simulink subsystem "Plant_d"  (R2024b)
settings: Solver=VariableStepAuto  StartTime=0.0  StopTime=10.0  RelTol=1e-3
undefined symbols (not defined in the file): body, DiscIntNeverNeededParam, wheels
settings Model: Creator=Marij  LastModifiedBy=marijn

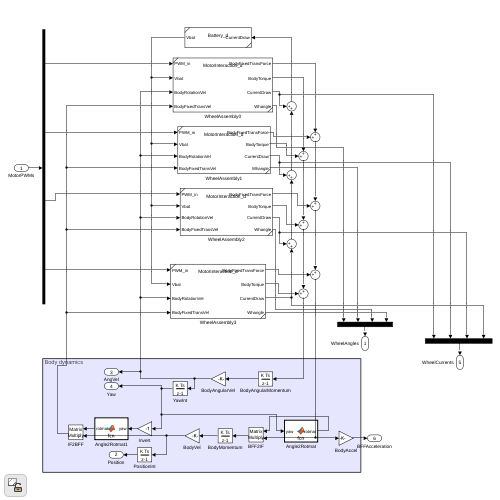
[thumbnail: Simulink's stored preview of the top-level diagram]
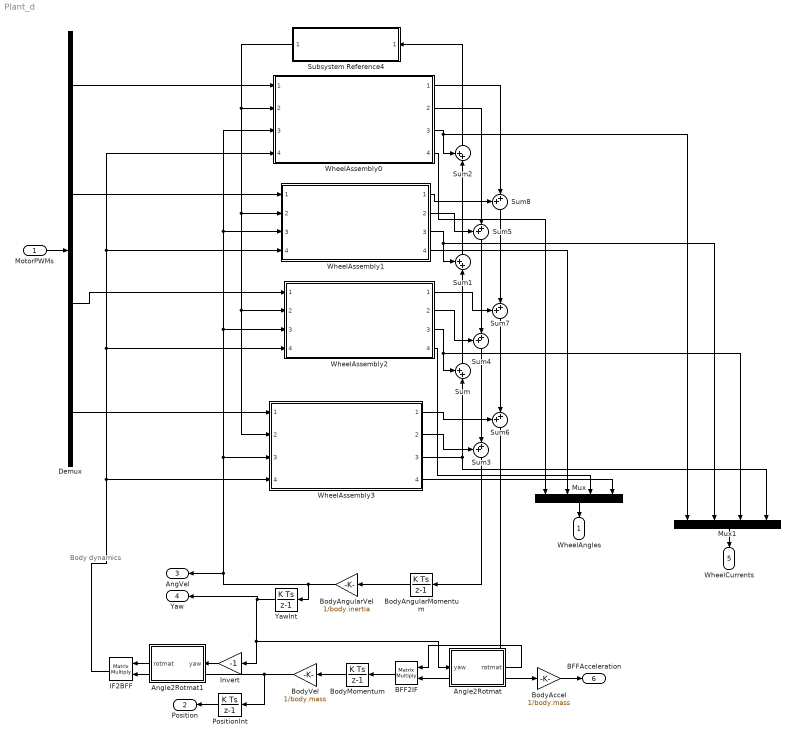
== system Plant_d ==
  note: Body dynamics
  MotorPWMs : Inport  PortDimensions=4
  Angle2Rotmat : MATLAB Function  TreatAsAtomicUnit=on
  Angle2Rotmat1 : MATLAB Function  TreatAsAtomicUnit=on
  BFF2IF : Product  Multiplication=Matrix(*)
  BodyAccel : Gain  Gain=1/body.mass
  BodyAngularMomentum : DiscreteIntegrator  SampleTime=0.0100000000000000002  ICPrevOutput=DiscIntNeverNeededParam  ICPrevScaledInput=DiscIntNeverNeededParam  mask(DiscretizedDiscreteIntegrator){}
      mask init:
      | %zoh
  BodyAngularVel : Gain  Gain=1/body.inertia
  BodyMomentum : DiscreteIntegrator  SampleTime=0.0100000000000000002  ICPrevOutput=DiscIntNeverNeededParam  ICPrevScaledInput=DiscIntNeverNeededParam  mask(DiscretizedDiscreteIntegrator){}
      mask init:
      | %zoh
  BodyVel : Gain  Gain=1/body.mass
  Demux : Demux
  IF2BFF : Product  Multiplication=Matrix(*)
  Invert : Gain  Gain=-1
  Mux : Mux
  Mux1 : Mux
  PositionInt : DiscreteIntegrator  SampleTime=0.0100000000000000002  ICPrevOutput=DiscIntNeverNeededParam  ICPrevScaledInput=DiscIntNeverNeededParam  mask(DiscretizedDiscreteIntegrator){}
      mask init:
      | %zoh
  Subsystem Reference4 : Subsystem  ReferencedSubsystem=Battery_d
  Sum{,1..8} (9 alike) : Sum  Inputs=++|
  WheelAssembly0 : Subsystem  ReferencedSubsystem=MotorInteraction_d  whangle=wheels.angles(1)
  WheelAssembly1 : Subsystem  ReferencedSubsystem=MotorInteraction_d  whangle=wheels.angles(2)
  WheelAssembly2 : Subsystem  ReferencedSubsystem=MotorInteraction_d  whangle=wheels.angles(3)
  WheelAssembly3 : Subsystem  ReferencedSubsystem=MotorInteraction_d  whangle=wheels.angles(4)
  YawInt : DiscreteIntegrator  SampleTime=0.0100000000000000002  ICPrevOutput=DiscIntNeverNeededParam  ICPrevScaledInput=DiscIntNeverNeededParam  mask(DiscretizedDiscreteIntegrator){}
      mask init:
      | %zoh
  WheelAngles : Outport  Unit=rad  PortDimensions=4
  Position : Outport  Port=2  Unit=m  PortDimensions=2
  AngVel : Outport  Port=3  Unit=rad/s  PortDimensions=1
  Yaw : Outport  Port=4  Unit=rad  PortDimensions=1
  WheelCurrents : Outport  Port=5  Unit=A  PortDimensions=4
  BFFAcceleration : Outport  Port=6
  wires:
  YawInt/1 -> Yaw/1, Angle2Rotmat/1(yaw), Invert/1
  BodyAccel/1 -> BFFAcceleration/1
  Subsystem Reference4/1 -> WheelAssembly0/2, WheelAssembly1/2, WheelAssembly2/2, WheelAssembly3/2
  Mux1/1 -> WheelCurrents/1
  Sum6/1 -> BodyAccel/1, BFF2IF/2
  Sum2/1 -> Subsystem Reference4/1
  WheelAssembly3/4 -> Mux/4
  WheelAssembly0/4 -> Mux/1
  Sum3/1 -> BodyAngularMomentum/1
  Angle2Rotmat1/1(rotmat) -> IF2BFF/1
  BodyMomentum/1 -> BodyVel/1
  BodyVel/1 -> PositionInt/1, IF2BFF/2
  IF2BFF/1 -> WheelAssembly2/4, WheelAssembly1/4, WheelAssembly0/4, WheelAssembly3/4
  Mux/1 -> WheelAngles/1
  BodyAngularMomentum/1 -> BodyAngularVel/1
  WheelAssembly2/2 -> Sum4/1
  WheelAssembly2/4 -> Mux/3
  WheelAssembly0/3 -> Mux1/1, Sum2/1
  PositionInt/1 -> Position/1
  MotorPWMs/1 -> Demux/1
  Sum/1 -> Sum1/2
  WheelAssembly1/3 -> Mux1/2, Sum1/1
  Sum1/1 -> Sum2/2
  Demux/3 -> WheelAssembly2/1
  Demux/4 -> WheelAssembly3/1
  WheelAssembly3/3 -> Mux1/4, Sum/2
  Demux/1 -> WheelAssembly0/1
  BodyAngularVel/1 -> YawInt/1, AngVel/1, WheelAssembly2/3, WheelAssembly1/3, WheelAssembly0/3, WheelAssembly3/3
  Sum8/1 -> Sum7/2
  Sum4/1 -> Sum3/2
  WheelAssembly1/4 -> Mux/2
  Angle2Rotmat/1(rotmat) -> BFF2IF/1
  BFF2IF/1 -> BodyMomentum/1
  WheelAssembly2/3 -> Mux1/3, Sum/1
  WheelAssembly1/1 -> Sum8/1
  WheelAssembly3/2 -> Sum3/1
  Invert/1 -> Angle2Rotmat1/1(yaw)
  WheelAssembly1/2 -> Sum5/1
  WheelAssembly0/1 -> Sum8/2
  Demux/2 -> WheelAssembly1/1
  WheelAssembly3/1 -> Sum6/1
  WheelAssembly2/1 -> Sum7/1
  Sum7/1 -> Sum6/2
  Sum5/1 -> Sum4/2
  WheelAssembly0/2 -> Sum5/2

== matlab function Plant_d/Angle2Rotmat ==
  data: yaw input; rotmat output
function rotmat = fcn(yaw)
rotmat = [cos(yaw), -sin(yaw); sin(yaw), cos(yaw)];

== matlab function Plant_d/Angle2Rotmat1 ==
  data: yaw input; rotmat output
function rotmat = fcn(yaw)
rotmat = [cos(yaw), -sin(yaw); sin(yaw), cos(yaw)];
